simulink model "MCU_Input"  (R2022b)
settings: Solver=FixedStepDiscrete  StartTime=0.0  StopTime=10.0  FixedStep=1e-4  RelTol=1e-3
values from neighbouring files (symbols this model uses):
  C_ADC_Acc1Offset_i32 = 0.0    [MCU_Input_Sldd.sldd]    (also in MCU_Input_Sldd_objects.m = myPackage.Parameter)
  C_ADC_BrakeOffset_i32 = 0.0    [MCU_Input_Sldd.sldd]    (also in MCU_Input_Sldd_objects.m = myPackage.Parameter)
  C_ADC_HSTempGain_f32 = 0.0    [MCU_Input_Sldd.sldd]    (also in MCU_Input_Sldd_objects.m = myPackage.Parameter)
  C_ADC_HSTempOffset_i32 = 0.0    [MCU_Input_Sldd.sldd]    (also in MCU_Input_Sldd_objects.m = myPackage.Parameter)
  C_ADC_IdcOffset_i32 = 0.0    [MCU_Input_Sldd.sldd]    (also in MCU_Input_Sldd_objects.m = myPackage.Parameter)
  C_ADC_IGBTTable_i16 = 0.0    [MCU_Input_Sldd.sldd]    (also in MCU_Input_Sldd_objects.m = myPackage.Parameter)
  C_ADC_IGBTTempGain_f32 = 0.0    [MCU_Input_Sldd.sldd]    (also in MCU_Input_Sldd_objects.m = myPackage.Parameter)
  C_ADC_IGBTTempOffset_i32 = 0.0    [MCU_Input_Sldd.sldd]    (also in MCU_Input_Sldd_objects.m = myPackage.Parameter)
  C_ADC_MotorTemp1Gain_f32 = 0.0    [MCU_Input_Sldd.sldd]    (also in MCU_Input_Sldd_objects.m = myPackage.Parameter)
  C_ADC_MotorTemp1Offset_i32 = 0.0    [MCU_Input_Sldd.sldd]    (also in MCU_Input_Sldd_objects.m = myPackage.Parameter)
  C_ADC_MotorTempTable_i16 = 0.0    [MCU_Input_Sldd.sldd]    (also in MCU_Input_Sldd_objects.m = myPackage.Parameter)
  C_ADC_P12VOffset_i32 = 0.0    [MCU_Input_Sldd.sldd]    (also in MCU_Input_Sldd_objects.m = myPackage.Parameter)
  C_ADC_P15VOffset_i32 = 0.0    [MCU_Input_Sldd.sldd]    (also in MCU_Input_Sldd_objects.m = myPackage.Parameter)
  C_ADC_P5VOffset_i32 = 0.0    [MCU_Input_Sldd.sldd]    (also in MCU_Input_Sldd_objects.m = myPackage.Parameter)
  C_DCCurrent_DrvCoeff_f32 = 0.0    [MCU_Input_Sldd.sldd]    (also in MCU_Input_Sldd_objects.m = myPackage.Parameter)
  C_DCCurrent_GenCoeff_f32 = 0.0    [MCU_Input_Sldd.sldd]    (also in MCU_Input_Sldd_objects.m = myPackage.Parameter)
  C_Encoder_CurrentAdder_f32 = 0.0    [MCU_Input_Sldd.sldd]    (also in MCU_Input_Sldd_objects.m = myPackage.Parameter)
  C_Encoder_WaitTime_f32 = 0.0    [MCU_Input_Sldd.sldd]    (also in MCU_Input_Sldd_objects.m = myPackage.Parameter)
  C_Input_EncErr_u8 = 0.0    [MCU_Input_Sldd.sldd]    (also in MCU_Input_Sldd_objects.m = myPackage.Parameter)
  C_Rotate_RotateBits_u8 = 0.0    [MCU_Input_Sldd.sldd]    (also in MCU_Input_Sldd_objects.m = myPackage.Parameter)
  C_Rotate_SetAngle_u16 = 0.0    [MCU_Input_Sldd.sldd]    (also in MCU_Input_Sldd_objects.m = myPackage.Parameter)
  C_Rotate_SetAngleFlg_u8 = 0.0    [MCU_Input_Sldd.sldd]    (also in MCU_Input_Sldd_objects.m = myPackage.Parameter)
  C_SelfCheck_AvgCntSet_u16 = 0.0    [MCU_Input_Sldd.sldd]    (also in MCU_Input_Sldd_objects.m = myPackage.Parameter)
  C_SelfCheck_DelayTimeSet_u16 = 0.0    [MCU_Input_Sldd.sldd]    (also in MCU_Input_Sldd_objects.m = myPackage.Parameter)
  C_SelfCheck_IaoffsetDownLimt_u16 = 0.0    [MCU_Input_Sldd.sldd]    (also in MCU_Input_Sldd_objects.m = myPackage.Parameter)
  C_SelfCheck_IaoffsetUpLimt_u16 = 0.0    [MCU_Input_Sldd.sldd]    (also in MCU_Input_Sldd_objects.m = myPackage.Parameter)
  C_SelfCheck_IboffsetDownLimt_u16 = 0.0    [MCU_Input_Sldd.sldd]    (also in MCU_Input_Sldd_objects.m = myPackage.Parameter)
  C_SelfCheck_IboffsetUpLimt_u16 = 0.0    [MCU_Input_Sldd.sldd]    (also in MCU_Input_Sldd_objects.m = myPackage.Parameter)
  C_SelfCheck_IcoffsetDownLimt_u16 = 0.0    [MCU_Input_Sldd.sldd]    (also in MCU_Input_Sldd_objects.m = myPackage.Parameter)
  C_SelfCheck_IcoffsetUpLimt_u16 = 0.0    [MCU_Input_Sldd.sldd]    (also in MCU_Input_Sldd_objects.m = myPackage.Parameter)
  C_SelfCheck_OffsetUnCal_u8 = 0.0    [MCU_Input_Sldd.sldd]    (also in MCU_Input_Sldd_objects.m = myPackage.Parameter)
undefined symbols (not defined in the file or in its folder): AB_SAMPLE, ABC_SAMPLE, AC_SAMPLE, ANALOG, BC_SAMPLE, cAgeingMode, cParaRecogMode, cVvvfOpenMode, ParamCfg_AdAcc1K_u16, ParamCfg_AdBrakeK_u16, ParamCfg_AdIaK_u16, ParamCfg_AdIbK_u16, ParamCfg_AdIcK_u16, ParamCfg_AdKeyK_u16, ParamCfg_AdP12vK_u16, ParamCfg_AdP15vK_u16, ParamCfg_AdP5vK_u16, ParamCfg_AdUdcK_u16, ParamCfg_AdVonK_u16, ParamCfg_Avgcnt_u16, ParamCfg_BaseCur_u16, ParamCfg_BaseUdc_u16, ParamCfg_CommandSource_u16, ParamCfg_MaxSpeed_u16, ParamCfg_MotorNp_u16, ParamCfg_PosInit_u16, ParamCfg_PowerMax_u16, ParamCfg_PwmFreqLow_u16, ParamCfg_RotateDir_u16, ParamCfg_RotateNp_u16, ParamCfg_SampleMode_u16, ParamCfg_SensorSpeed_u16, ParamCfg_SmoPllKi_u16, ParamCfg_SmoPllKp_u16, ParamCfg_Stage_u16, ParamCfg_ThetaGain_u16, ParamCfg_UdcDefValue_u16, POWER_ON, STANDBY
libraries: simulink x41, YS_UserDefined_Library x4
(part 4 of 5)

== stateflow chart MCU_Input/Input_100us/ETheta1/En/EncMode_Calc ==
  (default) -> (junction 169)
  (junction 169) -> (junction 171) [order 1] : [Standby==1]
  (junction 169) -> (junction 176) [order 2] : {
      | PosInput = Rotate_PosNew;
      | PosDelt = Rotate_PosDelt;
      | }
  (junction 171) -> (junction 175) : {
      | CurrentOutput=0;
      | WaitTime=0;
      | EAngle=0;
      | SysState=0;
      | PosInput=0;
      | PosDelt=0;
      | OverFlg=0;
      | }
  (junction 175) -> (junction 176)
  (junction 176) -> (junction 181)
  (junction 181) -> (junction 183) [order 2]
  (junction 183) -> (junction 185)
  (junction 181) -> (junction 25) [order 1] : [ParaRecogMode==1]
  (junction 25) -> (junction 26) [order 1] : [SysState == 0]
  (junction 25) -> (junction 29) [order 2]
  (junction 26) -> (junction 27) : {EAngle = 0}
  (junction 149) -> (junction 145) [order 1] : [TimeCnt >=20000 ]{TimeCnt=0;SysState=1}
  (junction 144) -> (junction 149) : {
      | CurrentOutput = GivenCurrent;
      | TimeCnt += 1;
      | }
  (junction 149) -> (junction 145) [order 2]
  (junction 27) -> (junction 144) [order 1] : [CurrentOutput >= GivenCurrent]
  (junction 145) -> (junction 28)
  (junction 27) -> (junction 28) [order 2] : {CurrentOutput +=CurAdder }
  (junction 28) -> (junction 32)
  (junction 29) -> (junction 30) [order 1] : [SysState == 1]
  (junction 29) -> (junction 33) [order 2]
  (junction 30) -> (junction 31) : {SysState = 2}
  (junction 31) -> (junction 32)
  (junction 32) -> (junction 36)
  (junction 33) -> (junction 34) [order 1] : [SysState == 2]
  (junction 33) -> (junction 37) [order 2]
  (junction 34) -> (junction 35) : {SysState = 3}
  (junction 35) -> (junction 36)
  (junction 36) -> (junction 40)
  (junction 37) -> (junction 38) [order 1] : [SysState == 3]
  (junction 37) -> (junction 69) [order 2]
  (junction 38) -> (junction 39) : {SysState = 4}
  (junction 39) -> (junction 40)
  (junction 40) -> (junction 75)
  (junction 69) -> (junction 71) [order 1] : [SysState == 4]
  (junction 69) -> (junction 78) [order 2]
  (junction 71) -> (junction 73) : {EAngle = 0}
  (junction 73) -> (junction 75) [order 1] : [WaitTime < WaitTimeOut]{WaitTime += 1}
  (junction 73) -> (junction 158) [order 2]
  (junction 158) -> (junction 75) [order 2]
  (junction 158) -> (junction 75) [order 1] : [abs(PosDelt)<2]
      | {
      | ZeroP = PosInput;
      | SysState = 5;
      | WaitTime = 0;
      | OverFlg = 1
      | }
  (junction 75) -> (junction 84)
  (junction 78) -> (junction 80) [order 1] : [SysState == 5]
  (junction 78) -> (junction 87) [order 2]
  (junction 80) -> (junction 82) : {CurrentOutput -=CurAdder }
  (junction 82) -> (junction 84) [order 2]
  (junction 82) -> (junction 84) [order 1] : [CurrentOutput <= 0]{CurrentOutput =0;SysState = 6}
  (junction 84) -> (junction 93)
  (junction 87) -> (junction 89) [order 1] : [SysState == 6]
  (junction 87) -> (junction 96) [order 2]
  (junction 89) -> (junction 91)
  (junction 91) -> (junction 93)
  (junction 93) -> (junction 132)
  (junction 132) -> (junction 96)
  (junction 96) -> (junction 137) : {CurOut = CurrentOutput *Idn }
  (junction 137) -> (junction 185)
  (junction 185) -> (junction 188)
  data: EAngle output single =0; CurAdder input single; SysState local double; CurrentOutput output single; GivenCurrent input single; ParaRecogMode input; TimeCnt local uint16 =0; Rotate_PosNew input; Rotate_PosDelt input; Standby input; WaitTimeOut input; WaitTime local single =0; ZeroP output single =0; OverFlg output uint8 =0; Idn input; CurOut output single =0; OverFlagOverWrite input; PosDelt local double; PosInput local double

== stateflow chart MCU_Input/Input_10ms/GPIO_Get_10ms/Read/GPIO_Signal_filter/Debounce1 ==
  (default) -> (junction 3)
  (junction 3) -> (junction 5) [order 1] : [XORresult  == 1]
  (junction 3) -> (junction 15) [order 2] : {Cnt = 0}
  (junction 5) -> (junction 8) : {Cnt = Cnt+1}
  (junction 8) -> (junction 11) [order 1] : [Cnt>=10]
  (junction 8) -> (junction 18) [order 2]
  (junction 11) -> (junction 13) : {Signal = OriginalSignal;
      | Cnt = 0}
  (junction 18) -> (junction 15)
  (junction 13) -> (junction 18)
  (junction 15) -> (junction 21)
  data: XORresult input; Signal output; OriginalSignal input =0; Cnt local =0

== stateflow chart MCU_Input/Input_10ms/GPIO_Get_10ms/Read/GPIO_Signal_filter/Debounce2 ==
  (default) -> (junction 3)
  (junction 3) -> (junction 5) [order 1] : [XORresult  == 1]
  (junction 3) -> (junction 15) [order 2] : {Cnt = 0}
  (junction 5) -> (junction 8) : {Cnt = Cnt+1}
  (junction 8) -> (junction 11) [order 1] : [Cnt>=10]
  (junction 8) -> (junction 18) [order 2]
  (junction 11) -> (junction 13) : {Signal = OriginalSignal;
      | Cnt = 0}
  (junction 18) -> (junction 15)
  (junction 13) -> (junction 18)
  (junction 15) -> (junction 21)
  data: XORresult input; Signal output; OriginalSignal input =0; Cnt local =0

== stateflow chart MCU_Input/Input_10ms/GPIO_Get_10ms/Read/GPIO_Signal_filter/Debounce ==
  (default) -> (junction 3)
  (junction 3) -> (junction 5) [order 1] : [XORresult  == 1]
  (junction 3) -> (junction 15) [order 2] : {Cnt = 0}
  (junction 5) -> (junction 8) : {Cnt = Cnt+1}
  (junction 8) -> (junction 11) [order 1] : [Cnt>=10]
  (junction 8) -> (junction 18) [order 2]
  (junction 11) -> (junction 13) : {Signal = OriginalSignal;
      | Cnt = 0}
  (junction 18) -> (junction 15)
  (junction 13) -> (junction 18)
  (junction 15) -> (junction 21)
  data: XORresult input; Signal output; OriginalSignal input =0; Cnt local =0

== stateflow chart MCU_Input/Input_10ms/GPIO_Get_10ms/Read/GPIO_Signal_filter/Debounce3 ==
  (default) -> (junction 3)
  (junction 3) -> (junction 5) [order 1] : [XORresult  == 1]
  (junction 3) -> (junction 15) [order 2] : {Cnt = 0}
  (junction 5) -> (junction 8) : {Cnt = Cnt+1}
  (junction 8) -> (junction 11) [order 1] : [Cnt>=10]
  (junction 8) -> (junction 18) [order 2]
  (junction 11) -> (junction 13) : {Signal = OriginalSignal;
      | Cnt = 0}
  (junction 18) -> (junction 15)
  (junction 13) -> (junction 18)
  (junction 15) -> (junction 21)
  data: XORresult input; Signal output; OriginalSignal input =0; Cnt local =0

== stateflow chart MCU_Input/Input_10ms/GPIO_Get_10ms/Read/GPIO_Signal_filter/Debounce4 ==
  (default) -> (junction 3)
  (junction 3) -> (junction 5) [order 1] : [XORresult  == 1]
  (junction 3) -> (junction 15) [order 2] : {Cnt = 0}
  (junction 5) -> (junction 8) : {Cnt = Cnt+1}
  (junction 8) -> (junction 11) [order 1] : [Cnt>=10]
  (junction 8) -> (junction 18) [order 2]
  (junction 11) -> (junction 13) : {Signal = OriginalSignal;
      | Cnt = 0}
  (junction 18) -> (junction 15)
  (junction 13) -> (junction 18)
  (junction 15) -> (junction 21)
  data: XORresult input; Signal output; OriginalSignal input =0; Cnt local =0

== stateflow chart MCU_Input/Input_10ms/GPIO_Get_10ms/Read/GPIO_Signal_filter/Debounce5 ==
  (default) -> (junction 3)
  (junction 3) -> (junction 5) [order 1] : [XORresult  == 1]
  (junction 3) -> (junction 15) [order 2] : {Cnt = 0}
  (junction 5) -> (junction 8) : {Cnt = Cnt+1}
  (junction 8) -> (junction 11) [order 1] : [Cnt>=10]
  (junction 8) -> (junction 18) [order 2]
  (junction 11) -> (junction 13) : {Signal = OriginalSignal;
      | Cnt = 0}
  (junction 18) -> (junction 15)
  (junction 13) -> (junction 18)
  (junction 15) -> (junction 21)
  data: XORresult input; Signal output; OriginalSignal input =0; Cnt local =0

== stateflow chart MCU_Input/Input_10ms/GPIO_Get_10ms/Read/GPIO_Signal_filter/Debounce6 ==
  (default) -> (junction 3)
  (junction 3) -> (junction 5) [order 1] : [XORresult  == 1]
  (junction 3) -> (junction 15) [order 2] : {Cnt = 0}
  (junction 5) -> (junction 8) : {Cnt = Cnt+1}
  (junction 8) -> (junction 11) [order 1] : [Cnt>=10]
  (junction 8) -> (junction 18) [order 2]
  (junction 11) -> (junction 13) : {Signal = OriginalSignal;
      | Cnt = 0}
  (junction 18) -> (junction 15)
  (junction 13) -> (junction 18)
  (junction 15) -> (junction 21)
  data: XORresult input; Signal output; OriginalSignal input =0; Cnt local =0

== stateflow chart MCU_Input/Input_10ms/GPIO_Get_10ms/Read/GPIO_Signal_filter/Debounce7 ==
  (default) -> (junction 3)
  (junction 3) -> (junction 5) [order 1] : [XORresult  == 1]
  (junction 3) -> (junction 15) [order 2] : {Cnt = 0}
  (junction 5) -> (junction 8) : {Cnt = Cnt+1}
  (junction 8) -> (junction 11) [order 1] : [Cnt>=10]
  (junction 8) -> (junction 18) [order 2]
  (junction 11) -> (junction 13) : {Signal = OriginalSignal;
      | Cnt = 0}
  (junction 18) -> (junction 15)
  (junction 13) -> (junction 18)
  (junction 15) -> (junction 21)
  data: XORresult input; Signal output; OriginalSignal input =0; Cnt local =0

== stateflow chart MCU_Input/Input_10ms/GPIO_Get_10ms/Read/GPIO_Signal_filter/Debounce8 ==
  (default) -> (junction 3)
  (junction 3) -> (junction 5) [order 1] : [XORresult  == 1]
  (junction 3) -> (junction 15) [order 2] : {Cnt = 0}
  (junction 5) -> (junction 8) : {Cnt = Cnt+1}
  (junction 8) -> (junction 11) [order 1] : [Cnt>=10]
  (junction 8) -> (junction 18) [order 2]
  (junction 11) -> (junction 13) : {Signal = OriginalSignal;
      | Cnt = 0}
  (junction 18) -> (junction 15)
  (junction 13) -> (junction 18)
  (junction 15) -> (junction 21)
  data: XORresult input; Signal output; OriginalSignal input =0; Cnt local =0

== stateflow chart MCU_Input/Input_100us/SelfCheck_100us/OffsetCal/IaOffsetCal ==
  state OffsetCalInit
  state OffsetCalFinish
    (default) -> (junction 37) : {StateOfOffsetcal = true}
  note: 增加PowerOn状态判断
      | 	1、只有在PowerOn状态才会做Offset计算
      | 	2、如果不是PowerOn状态则会退回初始化状态重新计算
      | 	3、只在PowerOn状态下完成一次Offset计算
  state OffsetCalRun
    (default) -> (junction 56) : {%持续清零
        | AvgCnt = 0;
        | ValSum = 0;}
  (default) -> OffsetCalInit
  OffsetCalFinish -> OffsetCalInit [commented out] : [PoweronState != 1 || StandbyState !=1]
  (junction 64) -> OffsetCalFinish [order 2] : {FlgOfEffectiveOffset = true}
  (junction 67) -> OffsetCalFinish : {FlgOfEffectiveOffset = false}
  (junction 61) -> OffsetCalFinish [commented out] : {FlgOfEffectiveOffset = false}
  OffsetCalInit -> (junction 41) : [PoweronState==1 || StandbyState ==1]
  OffsetCalRun -> OffsetCalInit [commented out] : [PoweronState != 1 || StandbyState != 1]
  (junction 41) -> OffsetCalRun : {ValSum = 0;
      | DelayCnt = 0;
      | AvgCnt = 0;
      | %OffsetTotalCnt = 0;
      | StateOfOffsetcal = false;
      | FlgOfEffectiveOffset = C_SelfCheck_OffsetUnCal_u8;
      | }
  (junction 64) -> (junction 67) [order 1] : [Offset > C_SelfCheck_IaoffsetUpLimt_u16...
      | || Offset < C_SelfCheck_IaoffsetDownLimt_u16]
  (junction 31) -> (junction 64) : {Offset = ValSum/AvgCntSet;}
  (junction 28) -> (junction 61) [commented out] : [OffsetTotalCnt > C_ADC_OffsetTotalCntSet_u16]
  OffsetCalRun -> (junction 74) [order 1] : [PoweronState==1]
  (junction 74) -> (junction 12) : [%源代码里有延迟172个tick在做累加的处理
      | DelayCnt < DelayTimeSet]
  (junction 12) -> (junction 14) : {DelayCnt = DelayCnt+1}
  (junction 28) -> (junction 31) : [AvgCnt >= AvgCntSet]
  OffsetCalRun -> (junction 28) [order 2] : {ValSum = ValSum + ADC_iNoOff;
      | AvgCnt = AvgCnt +1;}
  (junction 14) -> OffsetCalRun
  (junction 53) -> OffsetCalRun [commented out]
  OffsetCalRun -> (junction 45) [commented out] : [%判断Ia的ADC值如果一直超限允许值，就直接报错，不用再先求平均值然后和允许值做比较判断是否要报错
      | ADC_iNoOff > C_ADC_IaoffsetUpLimt_u16 || ADC_iNoOff<C_ADC_IaoffsetDownLimt_u16]
  (junction 45) -> (junction 49) [commented out] : [OffsetTotalCnt < C_ADC_OffsetTotalCntSet_u16]
  (junction 49) -> (junction 53) [commented out] : {OffsetTotalCnt ++}
  data: StandbyState input; PoweronState input; ADC_iNoOff input uint16; DelayTimeSet input uint16; AvgCntSet input uint16; DelayCnt local uint16 =0; ValSum local uint32 =0; AvgCnt local uint16 =0; Offset output single =0; StateOfOffsetcal output uint8 =0; OffsetTotalCnt local uint16 =0; FlgOfEffectiveOffset output uint8 =2; C_SelfCheck_OffsetUnCal_u8 parameter; C_SelfCheck_IaoffsetDownLimt_u16 parameter; C_SelfCheck_IaoffsetUpLimt_u16 parameter

== stateflow chart MCU_Input/Input_100us/SelfCheck_100us/OffsetCal/IbOffsetCal ==
  state OffsetCalInit
  state OffsetCalFinish
    (default) -> (junction 37) : {StateOfOffsetcal = true}
  note: 增加PowerOn状态判断
      | 	1、只有在PowerOn状态才会做Offset计算
      | 	2、如果不是PowerOn状态则会退回初始化状态重新计算
      | 	3、只在PowerOn状态下完成一次Offset计算
  state OffsetCalRun
    (default) -> (junction 56) : {
        | %持续清零
        | AvgCnt = 0;
        | ValSum = 0;}
  (default) -> OffsetCalInit
  OffsetCalFinish -> OffsetCalInit [commented out] : [PoweronState != 1]
  (junction 64) -> OffsetCalFinish [order 2] : {FlgOfEffectiveOffset = true}
  (junction 67) -> OffsetCalFinish : {FlgOfEffectiveOffset = false}
  (junction 61) -> OffsetCalFinish [commented out] : {FlgOfEffectiveOffset = false}
  OffsetCalInit -> (junction 41) : [PoweronState==1 || StandbyState ==1]
  OffsetCalRun -> OffsetCalInit [commented out] : [PoweronState != 1]
  (junction 41) -> OffsetCalRun : {ValSum = 0;
      | DelayCnt = 0;
      | AvgCnt = 0;
      | %OffsetTotalCnt = 0;
      | StateOfOffsetcal = false;
      | StateOfOffsetcal = false;
      | FlgOfEffectiveOffset = C_SelfCheck_OffsetUnCal_u8;}
  (junction 64) -> (junction 67) [order 1] : [Offset > C_SelfCheck_IboffsetUpLimt_u16...
      | || Offset < C_SelfCheck_IboffsetDownLimt_u16]
  (junction 31) -> (junction 64) : {Offset = ValSum/AvgCntSet;}
  (junction 28) -> (junction 61) [commented out] : [OffsetTotalCnt > C_ADC_OffsetTotalCntSet_u16]
  OffsetCalRun -> (junction 73) [order 1] : [PoweronState==1]
  (junction 73) -> (junction 12) : [%源代码里有延迟172个tick在做累加的处理
      | DelayCnt < DelayTimeSet]
  (junction 12) -> (junction 14) : {DelayCnt = DelayCnt+1}
  (junction 28) -> (junction 31) : [AvgCnt >= AvgCntSet]
  OffsetCalRun -> (junction 28) [order 2] : {ValSum = ValSum + ADC_iNoOff;
      | AvgCnt = AvgCnt +1;}
  (junction 14) -> OffsetCalRun
  (junction 53) -> OffsetCalRun [commented out]
  OffsetCalRun -> (junction 45) [commented out] : [%判断Ia的ADC值如果一直超限允许值，就直接报错，不用再先求平均值然后和允许值做比较判断是否要报错
      | ADC_iNoOff > C_ADC_IboffsetUpLimt_u16 || ADC_iNoOff<C_ADC_IboffsetDownLimt_u16]
  (junction 45) -> (junction 49) [commented out] : [OffsetTotalCnt < C_ADC_OffsetTotalCntSet_u16]
  (junction 49) -> (junction 53) [commented out] : {OffsetTotalCnt ++}
  data: StandbyState input; PoweronState input; ADC_iNoOff input uint16; DelayTimeSet input uint16; AvgCntSet input uint16; DelayCnt local uint16 =0; ValSum local uint32 =0; AvgCnt local uint16 =0; Offset output single =0; StateOfOffsetcal output uint8; OffsetTotalCnt local uint16 =0; FlgOfEffectiveOffset output uint8 =2; C_SelfCheck_OffsetUnCal_u8 parameter; C_SelfCheck_IboffsetUpLimt_u16 parameter; C_SelfCheck_IboffsetDownLimt_u16 parameter

== stateflow chart MCU_Input/Input_100us/SelfCheck_100us/OffsetCal/IcOffsetCal ==
  state OffsetCalInit
  state OffsetCalFinish
    (default) -> (junction 37) : {StateOfOffsetcal = true}
  note: 增加PowerOn状态判断
      | 	1、只有在PowerOn状态才会做Offset计算
      | 	2、如果不是PowerOn状态则会退回初始化状态重新计算
      | 	3、只在PowerOn状态下完成一次Offset计算
  state OffsetCalRun
    (default) -> (junction 56) : {
        | %持续清零
        | AvgCnt = 0;
        | ValSum = 0;}
  (default) -> OffsetCalInit
  OffsetCalFinish -> OffsetCalInit [commented out] : [PoweronState != 1]
  (junction 64) -> OffsetCalFinish [order 2] : {FlgOfEffectiveOffset = true}
  (junction 67) -> OffsetCalFinish : {FlgOfEffectiveOffset = false}
  (junction 61) -> OffsetCalFinish [commented out] : {FlgOfEffectiveOffset = false}
  OffsetCalInit -> (junction 41) : [PoweronState==1 || StandbyState ==1]
  OffsetCalRun -> OffsetCalInit [commented out] : [PoweronState != 1]
  (junction 41) -> OffsetCalRun : {ValSum = 0;
      | DelayCnt = 0;
      | AvgCnt = 0;
      | OffsetTotalCnt = 0;
      | StateOfOffsetcal = false;
      | StateOfOffsetcal = false;
      | FlgOfEffectiveOffset = C_SelfCheck_OffsetUnCal_u8;}
  (junction 64) -> (junction 67) [order 1] : [Offset > C_SelfCheck_IcoffsetUpLimt_u16...
      | || Offset < C_SelfCheck_IcoffsetDownLimt_u16]
  (junction 31) -> (junction 64) : {Offset = ValSum/AvgCntSet;}
  (junction 28) -> (junction 61) [commented out] : [OffsetTotalCnt > C_ADC_OffsetTotalCntSet_u16]
  OffsetCalRun -> (junction 73) [order 1] : [PoweronState==1]
  (junction 73) -> (junction 12) : [%源代码里有延迟172个tick在做累加的处理
      | DelayCnt < DelayTimeSet]
  (junction 12) -> (junction 14) : {DelayCnt = DelayCnt+1}
  (junction 28) -> (junction 31) : [AvgCnt >= AvgCntSet]
  OffsetCalRun -> (junction 28) [order 2] : {ValSum = ValSum + ADC_iNoOff;
      | AvgCnt = AvgCnt +1;}
  (junction 14) -> OffsetCalRun
  (junction 53) -> OffsetCalRun [commented out]
  OffsetCalRun -> (junction 45) [commented out] : [%判断Ia的ADC值如果一直超限允许值，就直接报错，不用再先求平均值然后和允许值做比较判断是否要报错
      | ADC_iNoOff > C_ADC_IcoffsetUpLimt_u16 || ADC_iNoOff<C_ADC_IcoffsetDownLimt_u16]
  (junction 45) -> (junction 49) [commented out] : [OffsetTotalCnt < C_ADC_OffsetTotalCntSet_u16]
  (junction 49) -> (junction 53) [commented out] : {OffsetTotalCnt ++}
  data: StandbyState input; PoweronState input; ADC_iNoOff input uint16; DelayTimeSet input uint16; AvgCntSet input uint16; DelayCnt local uint16 =0; ValSum local uint32 =0; AvgCnt local uint16 =0; Offset output single =0; StateOfOffsetcal output uint8 =0; OffsetTotalCnt local uint16 =0; FlgOfEffectiveOffset output uint8 =2; C_SelfCheck_OffsetUnCal_u8 parameter; C_SelfCheck_IcoffsetUpLimt_u16 parameter; C_SelfCheck_IcoffsetDownLimt_u16 parameter

== stateflow chart MCU_Input/Input_100us/Encoder_100us/Encoder_100us/EncCalibCal ==
  state Finish [commented out]
  state Normalize [commented out]
    en:
    if(Cnt<AvgCnt)
    SinAmplitude =AmpSin(SinDigitalValue);
    CosAmplitude = AmpCos(CosDigitalValue);
    %SinAmp = SinAmplitude;
    %CosAmp = CosAmplitude;
    SinSum = SinSum + SinDigitalValue;
    CosSum = CosSum + CosDigitalValue;
    Cnt = Cnt+1;
    else
    %求均值
    SinAverage = SinSum/(Cnt);
    CosAverage = CosSum/(Cnt);
    %求幅值倒数
    SinAmplitudeInverse = 1/SinAmplitude;
    CosAmplitudeInverse = 1/CosAmplitude;
    %更新参数，放大十倍写回
    SinAvg = SinAverage*10;
    CosAvg = CosAverage *10;
    SinAmp = SinAmplitude *10;
    CosAmp = CosAmplitude *10;
    SinValue = (SinDigitalValue-SinAverage)*SinAmplitudeInverse;
    CosValue = (CosDigitalValue - CosAverage)*CosAmplitudeInverse;
  state Compensate [commented out]
  state SinAmp = AmpSin(SinRaw) [function]
  state CosAmp = AmpCos(CosRaw) [function]
  (default) -> (junction 118) [commented out]
  (junction 118) -> Finish [commented out]
  (junction 118) -> Normalize [commented out] : [Calib_Stage == NORMALIZE]
  (junction 118) -> Compensate [commented out] : [Calib_Stage == COMPENSATE]
  Normalize -> Finish [commented out]
  (default) -> (junction 94) [commented out]
  (junction 108) -> (junction 117) [commented out] : [Cnt < AvgCnt]{
      | SinAmplitude =AmpSin(SinDigitalValue);
      | CosAmplitude = AmpCos(CosDigitalValue);
      |
      | %SinAmp = SinAmplitude;
      | %CosAmp = CosAmplitude;
      |
      | SinSum = SinSum + SinDigitalValue;
      | CosSum = CosSum + CosDigitalValue;
      | Cnt = Cnt+1;
      | }
  (junction 94) -> (junction 108) [commented out] : [Calib_Stage == NORMALIZE]
  (junction 108) -> (junction 117) [commented out]
  (junction 94) -> (junction 100) [commented out] : {SinSum = 0;
      | CosSum= 0;
      | Cnt = 0;
      | ToFinish = 0;
      | SinValue = (SinDigitalValue-SinAverage)*SinAmplitudeInverse;
      | CosValue = (CosDigitalValue - CosAverage)*CosAmplitudeInverse;
      | }
  (junction 117) -> (junction 95) [commented out] : {
      |     %求均值
      |     SinAverage = SinSum/(Cnt);
      |     CosAverage = CosSum/(Cnt);
      |
      |     %求幅值倒数
      |     SinAmplitudeInverse = 1/SinAmplitude;
      |     CosAmplitudeInverse = 1/CosAmplitude;
      |
      | %更新参数，放大十倍写回
      | SinAvg = SinAverage*10;
      | CosAvg = CosAverage *10;
      | SinAmp = SinAmplitude *10;
      | CosAmp = CosAmplitude *10;
      |
      | SinValue = (SinDigitalValue-SinAverage)*SinAmplitudeInverse;
      | CosValue = (CosDigitalValue - CosAverage)*CosAmplitudeInverse;
      | }
  (junction 100) -> (junction 112) [commented out]
  (junction 95) -> (junction 112) [commented out] : {SinSum = 0;
      | CosSum= 0;
      | Cnt = 0;
      | ToFinish = 0}
  (junction 112) -> (junction 107) [commented out]
  (default) -> (junction 151)
  (junction 151) -> (junction 153) [order 1] : [Calib_Stage == NORMALIZE && ToFinish!=1]
  (junction 151) -> (junction 166) [order 2]
  (junction 153) -> (junction 155)
  (junction 155) -> (junction 157) [order 1] : [Cnt < AvgCnt]
  (junction 155) -> (junction 161) [order 2] : {
      |     %求均值
      |     SinAverage = SinSum/(Cnt);
      |     CosAverage = CosSum/(Cnt);
      |
      |     %求幅值倒数
      |     SinAmplitudeInverse = 1/SinAmplitude;
      |     CosAmplitudeInverse = 1/CosAmplitude;
      |
      | %更新参数，放大十倍写回
      | SinAvg = SinAverage*10;
      | CosAvg = CosAverage *10;
      | SinAmp = SinAmplitude *10;
      | CosAmp = CosAmplitude *10;
      |
      | ToFinish = 1
      |
      | %SinValue = (SinDigitalValue-SinAverage)*SinAmplitudeInverse;
      | %CosValue = (CosDigitalValue - CosAverage)*CosAmplitudeInverse;
      | }
  (junction 157) -> (junction 159) : {
      | SinAmplitude =AmpSin(SinDigitalValue);
      | CosAmplitude = AmpCos(CosDigitalValue);
      |
      | %SinAmp = SinAmplitude;
      | %CosAmp = CosAmplitude;
      |
      | SinSum = SinSum + SinDigitalValue;
      | CosSum = CosSum + CosDigitalValue;
      | Cnt = Cnt+1;
      | }
  (junction 159) -> (junction 161)
  (junction 161) -> (junction 179)
  (junction 166) -> (junction 168) [order 1] : [Calib_Stage==COMPENSATE]
  (junction 166) -> (junction 170) [order 2] : %结束
      | {
      | Cnt=0;
      | SinSum=0
      | CosSum=0;
      | ToFinish=0;
      |
      | SinAverage = SinAvg*0.1;
      | CosAverage = CosAvg*0.1;
      |
      | SinAmplitudeInverse = 1/(SinAmp*0.1);
      | CosAmplitudeInverse = 1/(CosAmp*0.1);
      | }
  (junction 168) -> (junction 172) : {
      | SinAverage = SinAvg*0.1;
      | CosAverage = CosAvg*0.1;
      |
      | SinAmplitudeInverse = 1/(SinAmp*0.1);
      | CosAmplitudeInverse = 1/(CosAmp*0.1);
      | }
  (junction 172) -> (junction 174)
  (junction 174) -> (junction 176)
  (junction 176) -> (junction 170)
  (junction 179) -> (junction 176)
  (junction 170) -> (junction 182) : {
      | SinValue = (SinDigitalValue-SinAverage)*SinAmplitudeInverse;
      | CosValue = (CosDigitalValue - CosAverage)*CosAmplitudeInverse;
      | }
  data: SinRaw function_input uint16 size=1; SinAmp function_output single size=1; CosRaw function_input uint16 size=1; CosAmp function_output single; Calib_Stage input uint16; AvgCnt input uint16; CosDigitalValue input uint16; SinDigitalValue input uint16; CosValue output single; SinValue output single; Cnt local uint16 =0; CosSum local uint32 =0; SinSum local uint32 =0; COMPENSATE constant uint16 =2; NORMALIZE constant uint16 =1; SinAverage local single =0; CosAverage local single =0; CosAmplitudeInverse local single =0; SinAmplitudeInverse local single =0; CosAmplitude local single; SinAmplitude local single; CosAvg data_store_memory; SinAvg data_store_memory; SinAmp data_store_memory; CosAmp data_store_memory; ToFinish local uint8 =0

== stateflow chart MCU_Input/Input_100us/Encoder_100us/Encoder_100us/EncAngleCal/Chart ==
  state OutLimit = Limitation(In,Max,Min) [function]
  (default) -> (junction 5) : {
      | Err = Ref- Fdk;
      | Up = Kp *Err;
      | }
  (junction 5) -> (junction 11)
  (junction 11) -> (junction 15) [order 1] : [OutPreSat <= OutMax && OutPreSat >= OutMin]
  (junction 11) -> (junction 23) [order 2]
  (junction 15) -> (junction 18) : {Ui = Ui + (Ki * Up);}
  (junction 18) -> (junction 21)
  (junction 21) -> (junction 30)
  (junction 23) -> (junction 25) [order 1] : [OutPreSat > OutMax]
  (junction 25) -> (junction 27) [order 1] : [Err < 0 ]{Ui = Ui + (Ki * Up)}
  (junction 23) -> (junction 33) [order 2]
  (junction 25) -> (junction 27) [order 2]
  (junction 27) -> (junction 30)
  (junction 30) -> (junction 40)
  (junction 33) -> (junction 35) [order 1] : [OutPreSat < OutMin]
  (junction 35) -> (junction 37) [order 1] : [Err > 0 ]{Ui = Ui + (Ki * Up)}
  (junction 33) -> (junction 43) [order 2]
  (junction 35) -> (junction 37) [order 2]
  (junction 37) -> (junction 40)
  (junction 40) -> (junction 45)
  (junction 45) -> (junction 43)
  (junction 43) -> (junction 48) : {
      | OutPreSat = Up + Ui;
      | Out = Limitation(OutPreSat,OutMax,OutMin);
      | }
  data: In function_input; Max function_input; Min function_input; OutLimit function_output; Ref input single size=1; Fdk input single; Kp input single; Ki input single; OutMax input single size=1; OutMin input single size=1; Err local single size=1 =0; Up local single size=1; OutPreSat local single size=1; Ui local single; Out output single

== stateflow chart MCU_Input/Input_100us/ETheta/En/EncMode_Calc ==
  note: Do not put any code along
      | the transitions that run
      | down the right side!
  (default) -> (junction 25)
  (junction 25) -> (junction 26) [order 1] : [SysState == 0]
  (junction 25) -> (junction 29) [order 2]
  (junction 26) -> (junction 27) : {EAngle = 0}
  (junction 149) -> (junction 145) [order 1] : [TimeCnt >=20000 ]{TimeCnt=0;SysState=1}
  (junction 144) -> (junction 149) : {
      | CurrentOutput = GivenCurrent;
      | TimeCnt += 1;
      | }
  (junction 149) -> (junction 145) [order 2]
  (junction 27) -> (junction 144) [order 1] : [CurrentOutput >= GivenCurrent]
  (junction 145) -> (junction 28)
  (junction 27) -> (junction 28) [order 2] : {CurrentOutput +=CurAdder }
  (junction 28) -> (junction 32)
  (junction 29) -> (junction 30) [order 1] : [SysState == 1]
  (junction 29) -> (junction 33) [order 2]
  (junction 30) -> (junction 31) : {SysState = 2}
  (junction 31) -> (junction 32)
  (junction 32) -> (junction 36)
  (junction 33) -> (junction 34) [order 1] : [SysState == 2]
  (junction 33) -> (junction 37) [order 2]
  (junction 34) -> (junction 35) : {SysState = 3}
  (junction 35) -> (junction 36)
  (junction 36) -> (junction 40)
  (junction 37) -> (junction 38) [order 1] : [SysState == 3]
  (junction 37) -> (junction 69) [order 2]
  (junction 38) -> (junction 39) : {SysState = 4}
  (junction 39) -> (junction 40)
  (junction 40) -> (junction 75)
  (junction 69) -> (junction 71) [order 1] : [SysState == 4]
  (junction 69) -> (junction 78) [order 2]
  (junction 71) -> (junction 73) : {EAngle = 0}
  (junction 73) -> (junction 75) [order 1] : [WaitTime < WaitTimeOut]{WaitTime += 1}
  (junction 73) -> (junction 158) [order 2]
  (junction 158) -> (junction 75) [order 2]
  (junction 158) -> (junction 75) [order 1] : [abs(PosDelt)<2]
      | {
      | ZeroP = PosInput;
      | SysState = 5;
      | WaitTime = 0;
      | OverFlg = 1
      | }
  (junction 75) -> (junction 84)
  (junction 78) -> (junction 80) [order 1] : [SysState == 5]
  (junction 78) -> (junction 87) [order 2]
  (junction 80) -> (junction 82) : {CurrentOutput -=CurAdder }
  (junction 82) -> (junction 84) [order 2]
  (junction 82) -> (junction 84) [order 1] : [CurrentOutput <= 0]{CurrentOutput =0;SysState = 6}
  (junction 84) -> (junction 93)
  (junction 87) -> (junction 89) [order 1] : [SysState == 6]
  (junction 87) -> (junction 96) [order 2]
  (junction 89) -> (junction 91)
  (junction 91) -> (junction 93)
  (junction 93) -> (junction 132)
  (junction 132) -> (junction 96)
  (junction 96) -> (junction 137) : {CurOut = CurrentOutput *Idn }
  data: EAngle output single =0; CurAdder input single; SysState local double; CurrentOutput output single; GivenCurrent input single; TimeCnt local uint16 =0; PosInput input; PosDelt input; WaitTimeOut input; WaitTime local single =0; ZeroP output single =0; OverFlg output uint8 =0; Idn input; CurOut output single =0

== stateflow chart MCU_Input/Input_100us/Encoder_100us/Encoder_100us/EncCalibCal1 ==
  state Finish [commented out]
  state Normalize [commented out]
    en:
    if(Cnt<AvgCnt)
    SinAmplitude =AmpSin(SinDigitalValue);
    CosAmplitude = AmpCos(CosDigitalValue);
    %SinAmp = SinAmplitude;
    %CosAmp = CosAmplitude;
    SinSum = SinSum + SinDigitalValue;
    CosSum = CosSum + CosDigitalValue;
    Cnt = Cnt+1;
    else
    %求均值
    SinAverage = SinSum/(Cnt);
    CosAverage = CosSum/(Cnt);
    %求幅值倒数
    SinAmplitudeInverse = 1/SinAmplitude;
    CosAmplitudeInverse = 1/CosAmplitude;
    %更新参数，放大十倍写回
    SinAvg = SinAverage*10;
    CosAvg = CosAverage *10;
    SinAmp = SinAmplitude *10;
    CosAmp = CosAmplitude *10;
    SinValue = (SinDigitalValue-SinAverage)*SinAmplitudeInverse;
    CosValue = (CosDigitalValue - CosAverage)*CosAmplitudeInverse;
  state Compensate [commented out]
  state SinAmp = AmpSin(SinRaw) [function]
  state CosAmp = AmpCos(CosRaw) [function]
  (default) -> (junction 118) [commented out]
  (junction 118) -> Finish [commented out]
  (junction 118) -> Normalize [commented out] : [Calib_Stage == NORMALIZE]
  (junction 118) -> Compensate [commented out] : [Calib_Stage == COMPENSATE]
  Normalize -> Finish [commented out]
  (default) -> (junction 94) [commented out]
  (junction 108) -> (junction 117) [commented out] : [Cnt < AvgCnt]{
      | SinAmplitude =AmpSin(SinDigitalValue);
      | CosAmplitude = AmpCos(CosDigitalValue);
      |
      | %SinAmp = SinAmplitude;
      | %CosAmp = CosAmplitude;
      |
      | SinSum = SinSum + SinDigitalValue;
      | CosSum = CosSum + CosDigitalValue;
      | Cnt = Cnt+1;
      | }
  (junction 94) -> (junction 108) [commented out] : [Calib_Stage == NORMALIZE]
  (junction 108) -> (junction 117) [commented out]
  (junction 94) -> (junction 100) [commented out] : {SinSum = 0;
      | CosSum= 0;
      | Cnt = 0;
      | ToFinish = 0;
      | SinValue = (SinDigitalValue-SinAverage)*SinAmplitudeInverse;
      | CosValue = (CosDigitalValue - CosAverage)*CosAmplitudeInverse;
      | }
  (junction 117) -> (junction 95) [commented out] : {
      |     %求均值
      |     SinAverage = SinSum/(Cnt);
      |     CosAverage = CosSum/(Cnt);
      |
      |     %求幅值倒数
      |     SinAmplitudeInverse = 1/SinAmplitude;
      |     CosAmplitudeInverse = 1/CosAmplitude;
      |
      | %更新参数，放大十倍写回
      | SinAvg = SinAverage*10;
      | CosAvg = CosAverage *10;
      | SinAmp = SinAmplitude *10;
      | CosAmp = CosAmplitude *10;
      |
      | SinValue = (SinDigitalValue-SinAverage)*SinAmplitudeInverse;
      | CosValue = (CosDigitalValue - CosAverage)*CosAmplitudeInverse;
      | }
  (junction 100) -> (junction 112) [commented out]
  (junction 95) -> (junction 112) [commented out] : {SinSum = 0;
      | CosSum= 0;
      | Cnt = 0;
      | ToFinish = 0}
  (junction 112) -> (junction 107) [commented out]
  (default) -> (junction 151)
  (junction 151) -> (junction 153) [order 1] : [Calib_Stage == NORMALIZE && ToFinish!=1]
  (junction 151) -> (junction 166) [order 2]
  (junction 153) -> (junction 155)
  (junction 155) -> (junction 157) [order 1] : [Cnt < AvgCnt]
  (junction 155) -> (junction 161) [order 2] : {
      |     %求均值
      |     SinAverage = SinSum/(Cnt);
      |     CosAverage = CosSum/(Cnt);
      |
      |     %求幅值倒数
      |     SinAmplitudeInverse = 1/SinAmplitude;
      |     CosAmplitudeInverse = 1/CosAmplitude;
      |
      | %更新参数，放大十倍写回
      | SinAvg = SinAverage*10;
      | CosAvg = CosAverage *10;
      | SinAmp = SinAmplitude *10;
      | CosAmp = CosAmplitude *10;
      |
      | ToFinish = 1
      |
      | %SinValue = (SinDigitalValue-SinAverage)*SinAmplitudeInverse;
      | %CosValue = (CosDigitalValue - CosAverage)*CosAmplitudeInverse;
      | }
  (junction 157) -> (junction 159) : {
      | SinAmplitude =AmpSin(SinDigitalValue);
      | CosAmplitude = AmpCos(CosDigitalValue);
      |
      | %SinAmp = SinAmplitude;
      | %CosAmp = CosAmplitude;
      |
      | SinSum = SinSum + SinDigitalValue;
      | CosSum = CosSum + CosDigitalValue;
      | Cnt = Cnt+1;
      | }
  (junction 159) -> (junction 161)
  (junction 161) -> (junction 179)
  (junction 166) -> (junction 168) [order 1] : [Calib_Stage==COMPENSATE]
  (junction 166) -> (junction 170) [order 2] : %结束
      | {
      | Cnt=0;
      | SinSum=0
      | CosSum=0;
      | ToFinish=0;
      |
      | SinAverage = SinAvg*0.1;
      | CosAverage = CosAvg*0.1;
      |
      | SinAmplitudeInverse = 1/(SinAmp*0.1);
      | CosAmplitudeInverse = 1/(CosAmp*0.1);
      | }
  (junction 168) -> (junction 172) : {
      | SinAverage = SinAvg*0.1;
      | CosAverage = CosAvg*0.1;
      |
      | SinAmplitudeInverse = 1/(SinAmp*0.1);
      | CosAmplitudeInverse = 1/(CosAmp*0.1);
      | }
  (junction 172) -> (junction 174)
  (junction 174) -> (junction 176)
  (junction 176) -> (junction 170)
  (junction 179) -> (junction 176)
  (junction 170) -> (junction 182) : {
      | SinValue = (SinDigitalValue-SinAverage)*SinAmplitudeInverse;
      | CosValue = (CosDigitalValue - CosAverage)*CosAmplitudeInverse;
      | }
  data: SinRaw function_input uint16 size=1; SinAmp function_output single size=1; CosRaw function_input uint16 size=1; CosAmp function_output single; Calib_Stage input uint16; AvgCnt input uint16; CosDigitalValue input uint16; SinDigitalValue input uint16; CosValue output single; SinValue output single; Cnt local uint16 =0; CosSum local uint32 =0; SinSum local uint32 =0; COMPENSATE constant uint16 =2; NORMALIZE constant uint16 =1; SinAverage local single =0; CosAverage local single =0; CosAmplitudeInverse local single =0; SinAmplitudeInverse local single =0; CosAmplitude local single; SinAmplitude local single; CosAvg data_store_memory; SinAvg data_store_memory; SinAmp data_store_memory; CosAmp data_store_memory; ToFinish local uint8 =0

== stateflow chart MCU_Input/Input_100us/Encoder_100us/Encoder_100us/EncAngleCal/Chart1 ==
  (default) -> (junction 1)
  (junction 1) -> (junction 5) [order 1] : [FirstCalOver==0]
  (junction 1) -> (junction 11) [order 2] : {
      | CurrentAnglePu = AngleDelay
      | }
  (junction 5) -> (junction 8) : {
      | AnglePu = atan2(SinValue,CosValue)/PI;
      | CurrentAnglePu = AnglePu
      | FirstCalOver =1
      | }
  (junction 8) -> (junction 11)
  (junction 11) -> (junction 14)
  data: SinValue input single; CosValue input single; FirstCalOver local uint8 =0; PI constant single =3.14159265358979; CurrentAnglePu output single; AnglePu local single; AngleDelay input

== stateflow chart MCU_Input/Input_100us/Rotate_100us/RotateCalc/En/Chart ==
  state tmpPos = PosDirDispos(dir,pos,max_pos) [function]
  state tmpPos = PosLimit(pos,MaxPos) [function]
  (default) -> (junction 6)
  (junction 6) -> (junction 8) [order 1] : [Status ==START_SET  || SelfCheckNoOverFlag==1]
  (junction 6) -> (junction 27) [order 2]
  (junction 8) -> (junction 12) : {
      | Resolver_PosNew = EncCal_Angle;
      | PosStart = PosDirDispos(ParamCfg_RotateDir_u16,Resolver_PosNew,MaxPos);
      | PosNew = PosStart;
      | PosOld = PosNew;
      | Status = GET_DATA;
      |
      | }
  (junction 12) -> (junction 23)
  (junction 23) -> (junction 25)
  (junction 27) -> (junction 29) [order 1] : [Status ==GET_DATA]
  (junction 27) -> (junction 60) [order 2] : {Status = START_SET}
  (junction 29) -> (junction 31) : {PosOld = PosNew;
      | Resolver_PosNew = EncCal_Angle;
      | PosNew = PosDirDispos(ParamCfg_RotateDir_u16,Resolver_PosNew,MaxPos);
      | PosNew = PosLimit(PosNew,MaxPos);
      | PosDeltOld = PosDelt;
      | }
  (junction 25) -> (junction 57)
  (junction 31) -> (junction 49) [commented out] : [C_Rotate_SetAngleFlg_u8 == true]{PosDelt = C_Rotate_SetAngle_u16}
  (junction 45) -> (junction 38) [order 1] : [PosDelt> MaxBorder]{PosDelt = PosDelt - MaxPos}
  (junction 38) -> (junction 49)
  (junction 49) -> (junction 51) [order 1] : [AceCalc <ACE_CACL_DELAY]{AceCalc++}
  (junction 51) -> (junction 57) : {Status = GET_DATA}
  (junction 45) -> (junction 38) [order 2] : [PosDelt< -MaxBorder]{PosDelt = PosDelt + MaxPos}
  (junction 49) -> (junction 51) [order 2] : {PosAce = PosDelt-PosDeltOld}
  (junction 57) -> (junction 62)
  (junction 31) -> (junction 45) : {PosDelt = PosNew-PosOld}
  (junction 62) -> (junction 60)
  (junction 60) -> (junction 65)
  data: dir function_input uint16; pos function_input; max_pos function_input; tmpPos function_output; pos function_input; MaxPos function_input; tmpPos function_output; EncCal_Angle input uint16; MaxPos input uint16; PosStart output int32 =0; PosDelt output int16 =0; PosNew output int32 =0; Status local uint8 size=1 =1; START_SET constant uint8 =1; Resolver_PosNew local int32 size=1 =0; ParamCfg_RotateDir_u16 parameter; PosOld local int32; GET_DATA constant uint8 =2; PosDeltOld local int16 =0; C_Rotate_SetAngleFlg_u8 parameter; C_Rotate_SetAngle_u16 parameter; MaxBorder input; AceCalc local uint8 =0; ACE_CACL_DELAY constant uint8 =5; PosAce output int16; SelfCheckNoOverFlag input
